simulink model "extraquestlinear"  (R2015b)
settings: Solver=VariableStepAuto  StartTime=0.0  StopTime=10.0  RelTol=1e-3
values from neighbouring files (symbols this model uses):
  A = [ -1.3936    0.9744   -0.0019   -0.5349   -0.0071   -1.0562    0.4891 ... (first row only)    [jasdata.m]
  B = [ 0     0 ... (first row only)    [jasdata.m]
  C = [ 1     0     0     0     0     0     0 ... (first row only)    [jasdata.m]
  D = [ 0     0 ... (first row only)    [jasdata.m]
  Kf = 0.4*[1 1]    [design1.m]    (also in design2.m = 1.27*[1 1]; design3.m = 1.27*[1 1])
  T_f = 0.3    [design1.m]    (also in design2.m; design3.m = 0.03; sol5.m = 0.03)
undefined symbols (not defined in the file): Ctheta, L
settings Model: Creator=dell  LastModifiedBy=dell

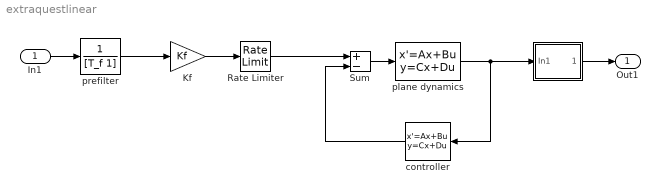
== system extraquestlinear ==
  In1 : Inport
  " " : Subsystem  mask(Matrix Gain){K=Ctheta}
      mask prompts: K "Gain matrix:"
      mask help: Matrix Gain.
      mask Help: Multiplies input vector by entered matrix to produce output vector (y=Au).
      mask Display: disp('Ctheta')
  Kf : Gain  Gain=Kf  SaturateOnIntegerOverflow=on  OutDataTypeStr=Inherit: Same as input  ParamDataTypeStr=Inherit: Same as input
  Rate Limiter : RateLimiter  SampleTimeMode=inherited
  Sum : Sum  Inputs=+-  SaturateOnIntegerOverflow=on  InputSameDT=on  OutDataTypeStr=Inherit: Same as first input
  controller : StateSpace  A=[]  B=[]  C=[]  D=K  X0=0  mask(Matrix gain){K=L}
      mask prompts: K "Gain matrix:"
      mask help: Matrix Gain:
      mask Help: Multiplies input vector by entered matrix to produce output vector.
      mask Display: disp('L')
  plane dynamics : StateSpace  A=A  B=B  C=C  D=D  X0=0
  prefilter : TransferFcn  Denominator=[T_f 1]
  Out1 : Outport
  wires:
  plane dynamics/1 -> " "/1(In1), controller/1
  Sum/1 -> plane dynamics/1
  controller/1 -> Sum/2
  prefilter/1 -> Kf/1
  Kf/1 -> Rate Limiter/1
  Rate Limiter/1 -> Sum/1
  In1/1 -> prefilter/1
  " "/1(Out1) -> Out1/1

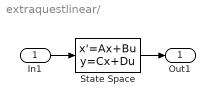
== system extraquestlinear/  ==
  In1 : Inport
  State Space : StateSpace  A=[]  B=[]  C=[]  D=K  X0=0
  Out1 : Outport
  wires:
  In1/1 -> State Space/1
  State Space/1 -> Out1/1
